simulink model "sawtoothsignal"  (R2023b)
settings: Solver=FixedStepDiscrete  StartTime=0.0  StopTime=10  RelTol=1e-3
values from neighbouring files (symbols this model uses):
  Fs = 1e6    (= 1000000)    [analyze_sin_signal.m]
undefined symbols (not defined in the file or in its folder): ip
libraries: plutoradiolib x1
settings Model: Creator=123  LastModifiedBy=yuezh

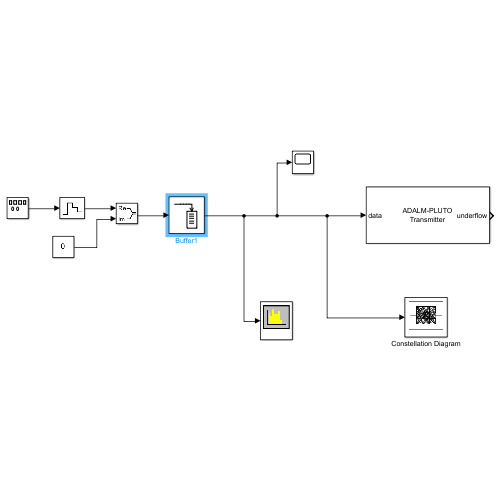
[thumbnail: Simulink's stored preview of the top-level diagram]
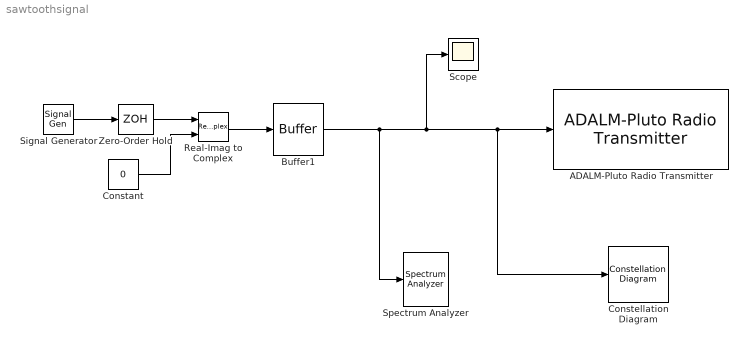
== system sawtoothsignal ==
  ADALM-Pluto Radio Transmitter : plutoradiolib/ADALM-Pluto Radio Transmitter  RadioID=ip:192.168.1.10  uri=ip:10.0.0.200  CenterFrequencySource=Dialog  CenterFrequency=2.2e9  GainSource=Dialog  Gain=-30  ChannelMapping=1  BasebandSampleRate=1e6  UnderflowOutputPort=on  ShowAdvancedProperties=off  UseCustomFilter=off  filtPathRates=[737280000 11520000 3840000 1920000 960000 240000]  filtCoefficients=[-192 82 85 -215 228 -102 -110 290 -318 145 160 -426 471 -215 -238 633 -697 318 349 -923 1009 -457 -498 1309 -1423 640 693 -1812 1959 -876 -945 2458 -2647 1180 1268 -3290 3534 -1572 -1688 4375 -4698 2091 2247 -5836 6284 -2807 -3031 7918 -8588 3870 4225 -11182 12324 -5662 -6330 17255 -19735 9507 11312 -33568 43355 -25227 -42139 305542 305542 -42139 -25227 43355 -33568 11312 9507 -19735 17255 -6330 -5662 12324 -11182 4225 3870 -8588 7918 -3031 -2807 6284 -5836 2247 2091 -4698 4375 -1688 -1572 3534 -3290 1268 1180 -2647 2458 -945 -876 1959 -1812 693 640 -1423 1309 -498 -457 1009 -923 349 318 -697 633 -238 -215 471 -426 160 145 -318 290 -110 -102 228 -215 85 82 -192]  filtCoefficientSize=128  filtDecimInterpFactor=4  filtGain=-12  filtRFBandwidth=18000000  filterConfigStruct=struct()  DataSourceSelect=Input Port  DDSTone1Freq=5e3  DDSTone2Freq=10e3  DDSTone1Scale=0.5  DDSTone2Scale=0.25  DataTimeout=Inf  FrequencyCorrection=0  ENSMPinControlMode=None  BISTLoopbackMode=Disabled  BISTToneInject=Disabled  BISTSignalGen=PRBS  BISTToneFreq=Fs/32  BISTToneLevel=0
  Buffer1 : Buffer  N=819200  OutputFrames=off
  Constant : Constant  Value=0  SampleTime=1/1e6
  Constellation Diagram : ConstellationDiagram  WindowPosition=[642.000000,50.000000,637.000000,305.000000,]  Visible=on  ScopeFrameLocation=window  XLimits=[-1.38,1.38]  YLimits=[-1.44,1.44]  ShowTrajectory=on  ColorFading=on
  Real-Imag to Complex : RealImagToComplex
  Scope : Scope
  Signal Generator : SignalGenerator  WaveForm=sawtooth  Amplitude=0.5  Frequency=200
  Spectrum Analyzer : SpectrumAnalyzer  WindowPosition=[642.000000,386.000000,637.000000,305.000000,]  Visible=on  ScopeFrameLocation=window  SampleRateSource=Property  SampleRate=1000000  PlotAsTwoSidedSpectrum=off  FrequencySpan=Start and stop frequencies  Span=2000  StartFrequency=0  StopFrequency=2000  RBWSource=Property  RBW=20  YLimits=[-35.64486972,18.7407484]
  Zero-Order Hold : ZeroOrderHold  SampleTime=1/1e6
  wires:
  Signal Generator/1 -> Zero-Order Hold/1
  Constant/1 -> Real-Imag to Complex/2
  Real-Imag to Complex/1 -> Buffer1/1
  Buffer1/1 -> Spectrum Analyzer/1, Scope/1, Constellation Diagram/1, ADALM-Pluto Radio Transmitter/1
  Zero-Order Hold/1 -> Real-Imag to Complex/1
